simulink model "Vehicle1D_TestModel"  (R2025a)
settings: Solver=daessc  StartTime=0.0  StopTime=300  RelTol=1e-3  AbsTol=1e-3
PreLoadFcn:
  | Vehicle1D_TestModelSetup
libraries: fl_lib x5, nesl_utility x3, simulink x3
settings Model: Creator=isaacito  LastModifiedBy=isaacito
settings SolverCC: AutoScaleAbsTol=off  AlgebraicLoopSolver=TrustRegion
settings DataIOCC: DSMLogging=off
settings OptimizationCC: ReuseModelBlockBuffer=off
settings DebuggingCC: UnconnectedInputMsg=warning  UnconnectedOutputMsg=warning  UnconnectedLineMsg=warning
settings ModelReferenceCC: EnableRefExpFcnMdlSchedulingChecks=on
settings RTWCC: GPUComputeCapability=3.5  DLArmComputeVersion=19.05
settings SimscapeCC: SimscapeLogType=all  SimscapeLogSimulationStatistics=on  SimscapeLogLimitData=off

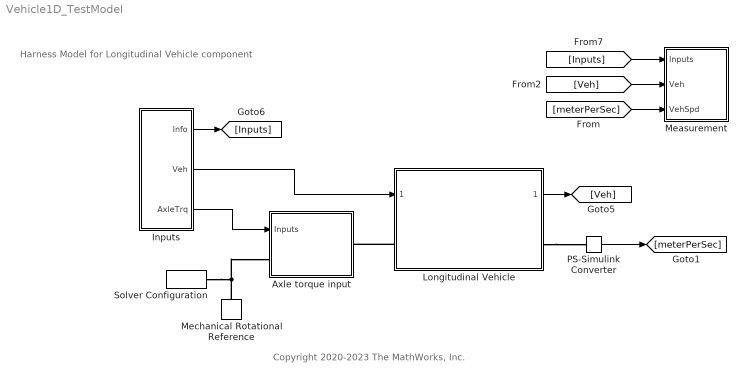
== system Vehicle1D_TestModel ==
  note: Harness Model for Longitudinal Vehicle component
  note: Copyright 2020-2023 The MathWorks, Inc.
  Axle torque input : Subsystem
  Inputs : Subsystem
  Longitudinal Vehicle : Subsystem  ReferencedSubsystem=Vehicle1D_Basic_refsub
      settings: OpenFcn=|
      | % Look under mask:
      | open_system(gcb, "force")
  Measurement : Subsystem
  Mechanical Rotational Reference : fl_lib/Mechanical/Rotational Elements/Mechanical Rotational Reference
  PS-Simulink Converter : nesl_utility/PS-Simulink Converter  PhysicalDomain=network_engine_domain  SubClassName=ps_output  LeftPortType=input  RightPortType=output  PseudoPeriodic=off  Frequencies=[]  VectorFormat=inherit  Unit=m/s  AffineConversion=off
  Solver Configuration : nesl_utility/Solver Configuration  PhysicalDomain=network_engine_domain  SubClassName=solver  LeftPortType=input  RightPortType=generic  Tones=[]  Harmonics=[]  SimulateNoise=off  Profile=off  UseLocalSampling=off  EnableSwitchedLinearOptims=on  FrequencyDomain=off  UseCCode=off  RelTol=0.001  AbsTol=1e-06  MinStep=1e-09  ToWorkspace=off  RevertToSquareIcSolve=off  NumHomotopyIterations=100  PhasorMode=off  PhasorModeNumHarmonics=1  ConsistencySolver=NEWTON_FTOL  IndexReductionMethod=DerivativeReplacement  DoDC=off  ResidualTolerance=1e-09  ConsistencyTolSource=GLOBAL  ConsistencyAbsTol=0.001  ConsistencyRelTol=0.001  ConsistencyTolFactor=0.001  UseLocalSolver=off  LocalSolverChoice=NE_BACKWARD_EULER_ADVANCER  ResolveIndetEquations=on  FunctionEvalNumThread=1  LocalSolverSampleTime=0.001  DoFixedCost=off  MaxNonlinIter=3  MaxModeIter=2  ComputeImpulses=off  ImpulseIterations=2  LinearAlgebra=auto  LinearAlgebraNumThread=0  EquationFormulation=NE_TIME_EF  DelaysMemoryBudget=1024  AutomaticFiltering=on  FilteringTimeConstant=0.001  PartitionStorageMethod=AS_NEEDED  PartitionMemoryBudget=1024  PartitionMethod=ROBUST  MultibodyUseLocalSolver=off  MultibodyLocalSolverChoice=ODE1  MultibodyLocalSolverSampleTime=0.001
      settings: AttributesFormatString=Local solver %<UseLocalSolver>
  wires:
  [Veh] -> Measurement/2(Veh)
  [Inputs] -> Measurement/1(Inputs)
  Longitudinal Vehicle/1 -> [Veh]
  Inputs/2(Veh) -> Longitudinal Vehicle/1
  Inputs/3(AxleTrq) -> Axle torque input/1(Inputs)
  Inputs/1(Info) -> [Inputs]
  PS-Simulink Converter/1 -> [meterPerSec]
  [meterPerSec] -> Measurement/3(VehSpd)
  connections:
  Longitudinal Vehicle/LConn1 -- Axle torque input/RConn1
  Mechanical Rotational Reference/LConn1 -- Axle torque input/LConn1 -- Solver Configuration/RConn1
  Longitudinal Vehicle/RConn1 -- PS-Simulink Converter/LConn1

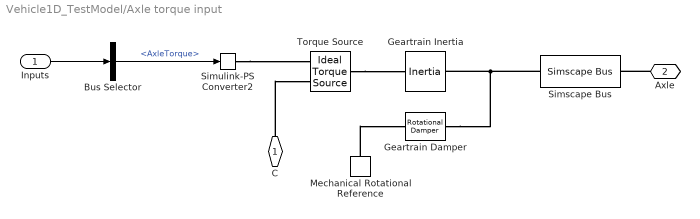
== system Vehicle1D_TestModel/Axle torque input ==
  Inputs : Inport
  Bus Selector : BusSelector  OutputSignals=AxleTorque
  Geartrain Damper : fl_lib/Mechanical/Rotational Elements/Rotational Damper  D=0.001 N*m*s/rad  w_specify=off  w_priority=None  w=0 rad/s  w_nominal_specify=off  w_nominal_value=1  w_nominal_unit=rad/s  t_specify=off  t_priority=None  t=0 N*m  t_nominal_specify=off  t_nominal_value=1  t_nominal_unit=N*m
  Geartrain Inertia : fl_lib/Mechanical/Rotational Elements/Inertia  inertia=1.35 kg*m^2  num_ports=foundation.enum.numPorts2.two  w_specify=on  w_priority=None  w=0 rpm  w_nominal_specify=off  w_nominal_value=1  w_nominal_unit=rad/s  t_specify=off  t_priority=None  t=0 N*m  t_nominal_specify=off  t_nominal_value=1  t_nominal_unit=N*m
      settings: InternalSimscapePortConfiguration="{\"Bottom\":[],\"Left\":[{\"id\":\"I\",\"label\":\"\",\"type\":\"foundation.mechanical.rotational.rotational\"}],\"Right\":[{\"id\":\"J\",\"label\":\"\",\"type\":\"foundation.mechanical.rotational.rotational\"}],\"Top\":[]}"
      settings: AttributesFormatString=|
      | %<inertia>
      | %<inertia_unit>
  Mechanical Rotational Reference : fl_lib/Mechanical/Rotational Elements/Mechanical Rotational Reference
  Simscape Bus : SimscapeBus  HierarchyStrings=AngSpd  ConnectionType=Bus: Bus_Rotational
      settings: AttributesFormatString=%<ConnectionType>
  Simulink-PS Converter2 : nesl_utility/Simulink-PS Converter  PhysicalDomain=network_engine_domain  SubClassName=ps_input  LeftPortType=input  RightPortType=output  PseudoPeriodic=off  Frequencies=[]  NoiseDistribution=none  NoiseParameters=[]  Unit=N*m  AffineConversion=off  FilteringAndDerivatives=filter  SimscapeFilterOrder=1  InputFilterTimeConstant=0.001  UdotUserProvided=0
  Torque Source : fl_lib/Mechanical/Mechanical Sources/Ideal Torque Source
  C : PMIOPort  Side=Left
  Axle : PMIOPort  Port=2  Side=Right
  wires:
  Inputs/1 -> Bus Selector/1
  Bus Selector/1 -> Simulink-PS Converter2/1  "<AxleTorque>"
  connections:
  C/RConn1 -- Torque Source/RConn2
  Simulink-PS Converter2/RConn1 -- Torque Source/RConn1
  Torque Source/LConn1 -- Geartrain Inertia/RConn1
  Simscape Bus/LConn1 -- Geartrain Damper/RConn1 -- Geartrain Inertia/LConn1
  Axle/RConn1 -- Simscape Bus/RConn1
  Mechanical Rotational Reference/LConn1 -- Geartrain Damper/LConn1

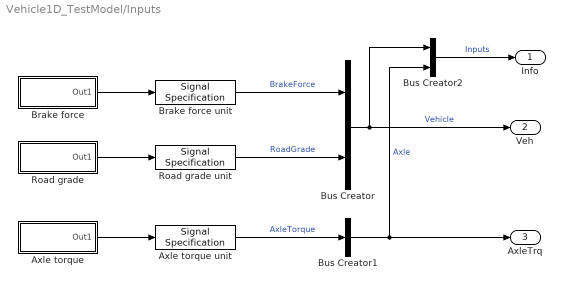
== system Vehicle1D_TestModel/Inputs ==
  Axle torque : Subsystem  mask(Continuous Multi-Step Signal){dataPoints=[0 10 0;30 100 400;140 200 900], deltaT=0.5}
      mask prompts: dataPoints "Data points"; deltaT "Interpolation step [s]"
      mask help:
      | This block generates a signal consisting of smoothly connected flat segments. Data points parameter takes an N-by-3 matrix where each row specifies a flat segment. First column and second column define start and end time of the segment, respectively. Third column defines the value of the segment. Second column can also be NaN to define a point value. Flat segments and point values are smoothly interpolated by Akima spline with the specified interpolation step.
      |
      | For example, a matrix [0 1 5; 3 nan 9; 6 8 7] for Data points defines a signal as follows. First row defines a flat segment from t=0 to t=1 of value 5. Second row defines a point at t=3 of value 9. Third row defines a flat segment from t=6 to t=8 of value 7.
      mask init:
      | sig = SignalDesigner("ContinuousMultiStep");
      | 
      | % Initialization function can access parameter names directly
      | sig.XYData = dataPoints;
      | sig.DeltaX = deltaT;
      | 
      | update(sig)
      | 
      | SignalSourceBlockCallback.setDataToLookupTableBlock( ...
      |   SignalObject = sig, ...
      |   PathToBlock = [gcb '/1-D Lookup Table']);
      mask DialogControl Control3 Prompt: horizontal spacer 1
      mask DialogControl Control4 Prompt: horizontal spacer 2
      mask DialogControl Control5 Prompt: horizontal spacer 3
      mask DialogControl PlotButton Prompt: Plot
      mask DialogControl PlotButton Callback: SignalSourceBlockCallback.plotContinuousMultiStep(gcb);
      mask Display: disp("Continuous" + newline + "Multi-Step")
  Axle torque unit : SignalSpecification  Unit=N*m
  Brake force : Subsystem  mask(Continuous Multi-Step Signal){dataPoints=[0 1 0], deltaT=0.5}
      mask prompts: dataPoints "Data points"; deltaT "Interpolation step [s]"
      mask help:
      | This block generates a signal consisting of smoothly connected flat segments. Data points parameter takes an N-by-3 matrix where each row specifies a flat segment. First column and second column define start and end time of the segment, respectively. Third column defines the value of the segment. Second column can also be NaN to define a point value. Flat segments and point values are smoothly interpolated by Akima spline with the specified interpolation step.
      |
      | For example, a matrix [0 1 5; 3 nan 9; 6 8 7] for Data points defines a signal as follows. First row defines a flat segment from t=0 to t=1 of value 5. Second row defines a point at t=3 of value 9. Third row defines a flat segment from t=6 to t=8 of value 7.
      mask init: same as Vehicle1D_TestModel/Inputs/Axle torque
      mask DialogControl Control3 Prompt: horizontal spacer 1
      mask DialogControl Control4 Prompt: horizontal spacer 2
      mask DialogControl Control5 Prompt: horizontal spacer 3
      mask DialogControl PlotButton Prompt: Plot
      mask DialogControl PlotButton Callback: SignalSourceBlockCallback.plotContinuousMultiStep(gcb);
      mask Display: disp("Continuous" + newline + "Multi-Step")
  Brake force unit : SignalSpecification  Unit=N
  Bus Creator : BusCreator  Inputs=2
  Bus Creator1 : BusCreator  Inputs=1
  Bus Creator2 : BusCreator  Inputs=2
  Road grade : Subsystem  mask(Continuous Multi-Step Signal){dataPoints=[0 1 0], deltaT=0.5}
      mask prompts: dataPoints "Data points"; deltaT "Interpolation step [s]"
      mask help:
      | This block generates a signal consisting of smoothly connected flat segments. Data points parameter takes an N-by-3 matrix where each row specifies a flat segment. First column and second column define start and end time of the segment, respectively. Third column defines the value of the segment. Second column can also be NaN to define a point value. Flat segments and point values are smoothly interpolated by Akima spline with the specified interpolation step.
      |
      | For example, a matrix [0 1 5; 3 nan 9; 6 8 7] for Data points defines a signal as follows. First row defines a flat segment from t=0 to t=1 of value 5. Second row defines a point at t=3 of value 9. Third row defines a flat segment from t=6 to t=8 of value 7.
      mask init: same as Vehicle1D_TestModel/Inputs/Axle torque
      mask DialogControl Control3 Prompt: horizontal spacer 1
      mask DialogControl Control4 Prompt: horizontal spacer 2
      mask DialogControl Control5 Prompt: horizontal spacer 3
      mask DialogControl PlotButton Prompt: Plot
      mask DialogControl PlotButton Callback: SignalSourceBlockCallback.plotContinuousMultiStep(gcb);
      mask Display: disp("Continuous" + newline + "Multi-Step")
  Road grade unit : SignalSpecification  Unit=%
  Info : Outport
  Veh : Outport  Port=2
  AxleTrq : Outport  Port=3  Unit=N*m
  wires:
  Brake force/1(Out1) -> Brake force unit/1
  Road grade/1(Out1) -> Road grade unit/1
  Bus Creator/1 -> Bus Creator2/1, Veh/1  "Vehicle"
  Axle torque/1(Out1) -> Axle torque unit/1
  Brake force unit/1 -> Bus Creator/1  "BrakeForce"
  Road grade unit/1 -> Bus Creator/2  "RoadGrade"
  Axle torque unit/1 -> Bus Creator1/1  "AxleTorque"
  Bus Creator1/1 -> Bus Creator2/2, AxleTrq/1  "Axle"
  Bus Creator2/1 -> Info/1  "Inputs"

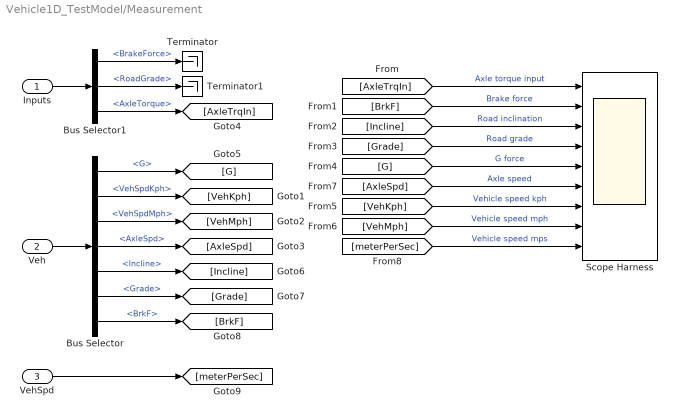
== system Vehicle1D_TestModel/Measurement ==
  Inputs : Inport
  Veh : Inport  Port=2
  VehSpd : Inport  Port=3  Unit=m/s
  Bus Selector : BusSelector  OutputSignals=G,VehSpdKph,VehSpdMph,AxleSpd,Incline,Grade,BrkF
  Bus Selector1 : BusSelector  OutputSignals=Vehicle.BrakeForce,Vehicle.RoadGrade,Axle.AxleTorque
  Scope Harness : Scope  NumInputPorts=9
      settings: ActiveDisplayYMinimum=-112.5  ActiveDisplayYMaximum=1012.5
  Terminator : Terminator
  Terminator1 : Terminator
  wires:
  Veh/1 -> Bus Selector/1
  Bus Selector/1 -> [G]  "<G>"
  Bus Selector/2 -> [VehKph]  "<VehSpdKph>"
  Bus Selector/3 -> [VehMph]  "<VehSpdMph>"
  Bus Selector/4 -> [AxleSpd]  "<AxleSpd>"
  Bus Selector/5 -> [Incline]  "<Incline>"
  Bus Selector/6 -> [Grade]  "<Grade>"
  Bus Selector/7 -> [BrkF]  "<BrkF>"
  [Grade] -> Scope Harness/4  "Road grade"
  [Incline] -> Scope Harness/3  "Road inclination"
  [G] -> Scope Harness/5  "G force"
  [BrkF] -> Scope Harness/2  "Brake force"
  [AxleTrqIn] -> Scope Harness/1  "Axle torque input"
  Inputs/1 -> Bus Selector1/1
  Bus Selector1/1 -> Terminator/1  "<BrakeForce>"
  Bus Selector1/2 -> Terminator1/1  "<RoadGrade>"
  Bus Selector1/3 -> [AxleTrqIn]  "<AxleTorque>"
  VehSpd/1 -> [meterPerSec]
  [AxleSpd] -> Scope Harness/6  "Axle speed"
  [VehKph] -> Scope Harness/7  "Vehicle speed kph"
  [VehMph] -> Scope Harness/8  "Vehicle speed mph"
  [meterPerSec] -> Scope Harness/9  "Vehicle speed mps"

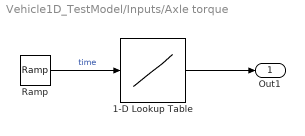
== system Vehicle1D_TestModel/Inputs/Axle torque ==
  1-D Lookup Table : Lookup_n-D  NumberOfTableDimensions=1  BreakpointsForDimension1="[0            10          10.5            11          11.5            12          12.5            13          13.5            14          14.5            15          15.5            16          16.5            17          17.5            18          18.5            19          19.5            20          20.5            21          21.5            22          22.5            23          23.5            24          24.5            25          25.5            26          26.5            27          27.5            28          28.5            29          29.5            30           100         100.5           101         101.5           102         102.5           103         103.5           104         104.5           105         105.5           106         106.5           107         107.5           108         108.5           109         109.5           110         110.5           111         111.5           112         112.5           113         113.5           114         114.5           115         115.5           116         116.5           117         117.5           118         118.5           119         119.5           120         120.5           121         121.5           122         122.5           123         123.5           124         124.5           125         125.5           126         126.5           127         127.5           128         128.5           129         129.5           130         130.5           131         131.5           132         132.5           133         133.5           134         134.5           135         135.5           136         136.5           137         137.5           138         138.5           139         139.5           140           200]"  Table="[0             0        0.7375           2.9        6.4125          11.2       17.1875          24.3       32.4625          41.6       51.6375          62.5       74.1125          86.4       99.2875         112.7      126.5625         140.8      155.3375         170.1      185.0125           200      214.9875         229.9      244.6625         259.2      273.4375         287.3      300.7125         313.6      325.8875         337.5      348.3625         358.4      367.5375         375.7      382.8125         388.8      393.5875         397.1      399.2625           400           400      400.2324      400.9219      402.0566       403.625      405.6152      408.0156      410.8145           414      417.5605      421.4844      425.7598       430.375      435.3184      440.5781      446.1426           452      458.1387      464.5469      471.2129       478.125      485.2715      492.6406      500.2207           508      515.9668      524.1094       532.416       540.875      549.4746      558.2031      567.0488           576      585.0449      594.1719      603.3691       612.625      621.9277      631.2656       640.627           650       659.373      668.7344      678.0723       687.375      696.6309      705.8281      714.9551           724      732.9512      741.7969      750.5254       759.125       767.584      775.8906      784.0332           792      799.7793      807.3594      814.7285       821.875      828.7871      835.4531      841.8613           848      853.8574      859.4219      864.6816       869.625      874.2402      878.5156      882.4395           886      889.1855      891.9844      894.3848       896.375      897.9434      899.0781      899.7676           900           900]"  InternalRulePriority=Speed  RndMeth=Simplest
  Ramp : simulink/Sources/Ramp  slope=1  start=0  InitialOutput=0
      settings: AttributesFormatString=|
      | Slope: %<slope>
      | Start time: %<start>
      | Initial output: %<InitialOutput>
  Out1 : Outport
  wires:
  Ramp/1 -> 1-D Lookup Table/1  "time"
  1-D Lookup Table/1 -> Out1/1

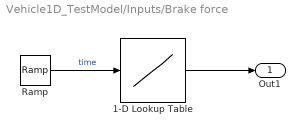
== system Vehicle1D_TestModel/Inputs/Brake force ==
  1-D Lookup Table : Lookup_n-D  NumberOfTableDimensions=1  BreakpointsForDimension1="[0  1]"  Table="[0  0]"  InternalRulePriority=Speed  RndMeth=Simplest
  Ramp : simulink/Sources/Ramp  slope=1  start=0  InitialOutput=0
      settings: AttributesFormatString=|
      | Slope: %<slope>
      | Start time: %<start>
      | Initial output: %<InitialOutput>
  Out1 : Outport
  wires:
  Ramp/1 -> 1-D Lookup Table/1  "time"
  1-D Lookup Table/1 -> Out1/1

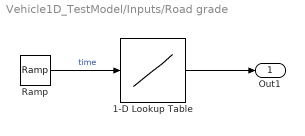
== system Vehicle1D_TestModel/Inputs/Road grade ==
  1-D Lookup Table : Lookup_n-D  NumberOfTableDimensions=1  BreakpointsForDimension1="[0  1]"  Table="[0  0]"  InternalRulePriority=Speed  RndMeth=Simplest
  Ramp : simulink/Sources/Ramp  slope=1  start=0  InitialOutput=0
      settings: AttributesFormatString=|
      | Slope: %<slope>
      | Start time: %<start>
      | Initial output: %<InitialOutput>
  Out1 : Outport
  wires:
  Ramp/1 -> 1-D Lookup Table/1  "time"
  1-D Lookup Table/1 -> Out1/1
